simulink model "ex_06_model"  (R2014a)
settings: Solver=ode45  StartTime=0.0  StopTime=10.0  RelTol=1e-3
values from neighbouring files (symbols this model uses):
  G = 0    [ex_06_init.m]
  x = -(1/J) * (a + (K^2/R))    (= -20.4)    [ex_06_init.m]
  y = (K/(J*R))    (= 400)    [ex_06_init.m]
  z = -(1/J)    (= -4000)    [ex_06_init.m]
settings Model: Creator=Nino  LastModifiedBy=Nino

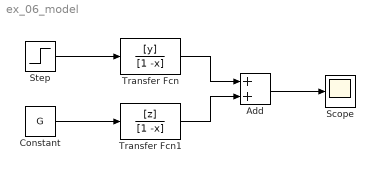
== system ex_06_model ==
  Add : Sum
  Constant : Constant  Value=G
  Scope : Scope
  Step : Step  After=10  SampleTime=0
  Transfer Fcn : TransferFcn  Numerator=[y]  Denominator=[1 -x]
  Transfer Fcn1 : TransferFcn  Numerator=[z]  Denominator=[1 -x]
  wires:
  Transfer Fcn/1 -> Add/1
  Transfer Fcn1/1 -> Add/2
  Add/1 -> Scope/1
  Step/1 -> Transfer Fcn/1
  Constant/1 -> Transfer Fcn1/1
